simulink model "zad_3_sch_2022a"  (R2022a)
settings: Solver=FixedStepAuto  StartTime=0.0  StopTime=15  FixedStep=0.0001  RelTol=1e-3
InitFcn:
  | Kp=-50
  | Ti=10
  | Td=.4
values from neighbouring files (symbols this model uses):
  a21 = 1/(2*m)*x30^2*FemP1/FemP2^2*exp(-x10/FemP2)    [zad_3.m]
  a23 = -1/(m)*x30*FemP1/FemP2*exp(-x10/FemP2)    [zad_3.m]
  a31 = 1/f1*exp(x10/f2)*(ki*u10+ci-x30)    [zad_3.m]
  a33 = -f2/f1*exp(x10/f2)    [zad_3.m]
  b31 = ki*f2/f1*exp(x10/f2)    [zad_3.m]
  g = 9.81    [zad_3.m]
  xd = d-bd    (= 0.0192)    [zad_3.m]
settings Model: Creator=MPatr  LastModifiedBy=MPatr
settings ModelReferenceCC: EnableRefExpFcnMdlSchedulingChecks=off
settings RTWCC: Description=Generic Real-Time Target

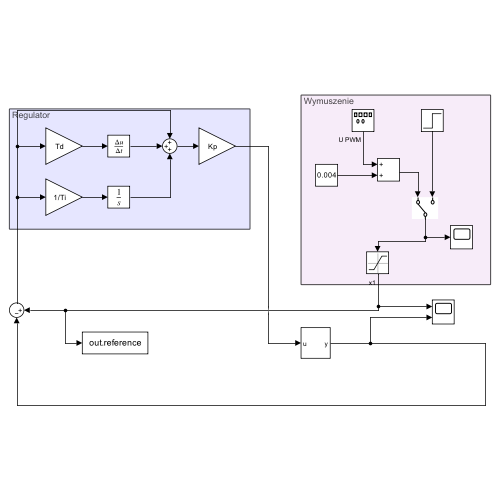
[thumbnail: Simulink's stored preview of the top-level diagram]
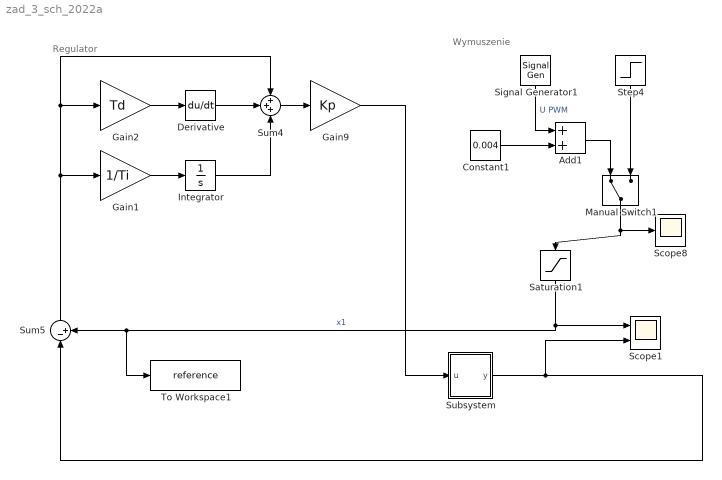
== system zad_3_sch_2022a ==
  note: Wymuszenie
  note: Regulator
  Add1 : Sum
  Constant1 : Constant  Value=0.004
  Derivative : Derivative
  Gain1 : Gain  Gain=1/Ti
  Gain2 : Gain  Gain=Td
  Gain9 : Gain  Gain=Kp
  Integrator : Integrator
  Manual Switch1 : ManualSwitch
  Saturation1 : Saturate  UpperLimit=1  LowerLimit=0
  Scope1 : Scope  NumInputPorts=2
  Scope8 : Scope
  Signal Generator1 : SignalGenerator  Amplitude=.002  Units=rad/sec
  Step4 : Step  Time=0  After=0.003  SampleTime=0
  Subsystem : Subsystem
  Sum4 : Sum  Inputs=+++
  Sum5 : Sum  Inputs=|-+
  To Workspace1 : ToWorkspace  VariableName=reference  SaveFormat=Structure With Time  SampleTime=-1
  wires:
  Saturation1/1 -> Scope1/1, To Workspace1/1, Sum5/2  "x1"
  Signal Generator1/1 -> Add1/1  "U PWM"
  Constant1/1 -> Add1/2
  Add1/1 -> Manual Switch1/1
  Manual Switch1/1 -> Scope8/1, Saturation1/1
  Step4/1 -> Manual Switch1/2
  Sum5/1 -> Gain2/1, Sum4/1, Gain1/1
  Gain1/1 -> Integrator/1
  Integrator/1 -> Sum4/3
  Sum4/1 -> Gain9/1
  Derivative/1 -> Sum4/2
  Gain2/1 -> Derivative/1
  Gain9/1 -> Subsystem/1(u)
  Subsystem/1(y) -> Scope1/2, Sum5/1

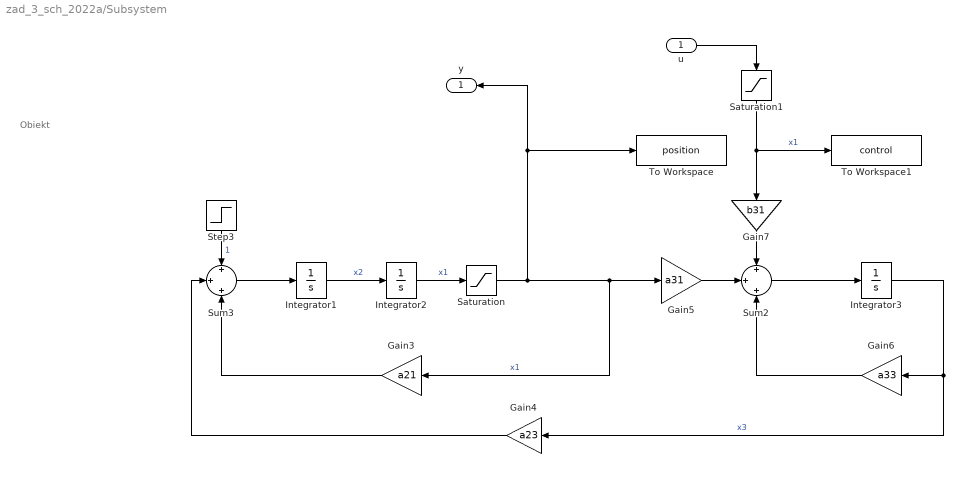
== system zad_3_sch_2022a/Subsystem ==
  note: Obiekt
  u : Inport
  Gain3 : Gain  Gain=a21
  Gain4 : Gain  Gain=a23
  Gain5 : Gain  Gain=a31
  Gain6 : Gain  Gain=a33
  Gain7 : Gain  Gain=b31
  Integrator1 : Integrator
  Integrator2 : Integrator  InitialCondition=xd
  Integrator3 : Integrator
  Saturation : Saturate  UpperLimit=xd  LowerLimit=0
  Saturation1 : Saturate  UpperLimit=1  LowerLimit=0
  Step3 : Step  Time=0  After=g  SampleTime=0
  Sum2 : Sum  Inputs=+|+|+
  Sum3 : Sum  Inputs=+|+|+
  To Workspace : ToWorkspace  VariableName=position  SaveFormat=Structure With Time  SampleTime=-1
  To Workspace1 : ToWorkspace  VariableName=control  SaveFormat=Structure With Time  SampleTime=-1
  y : Outport
  wires:
  Step3/1 -> Sum3/1  "1"
  Sum3/1 -> Integrator1/1
  Integrator2/1 -> Saturation/1  "x1"
  Saturation/1 -> y/1, To Workspace/1, Gain5/1, Gain3/1  "x1"
  Integrator1/1 -> Integrator2/1  "x2"
  Integrator3/1 -> Gain6/1, Gain4/1  "x3"
  Gain4/1 -> Sum3/2
  Sum2/1 -> Integrator3/1
  Gain5/1 -> Sum2/2
  Gain7/1 -> Sum2/1
  Gain6/1 -> Sum2/3
  Gain3/1 -> Sum3/3
  u/1 -> Saturation1/1
  Saturation1/1 -> To Workspace1/1, Gain7/1  "x1"
